simulink model "test_charti"  (R2014a)
settings: Solver=ode45  StartTime=0.0  StopTime=10.0  RelTol=1e-3
settings Model: Creator=simon  LastModifiedBy=simon

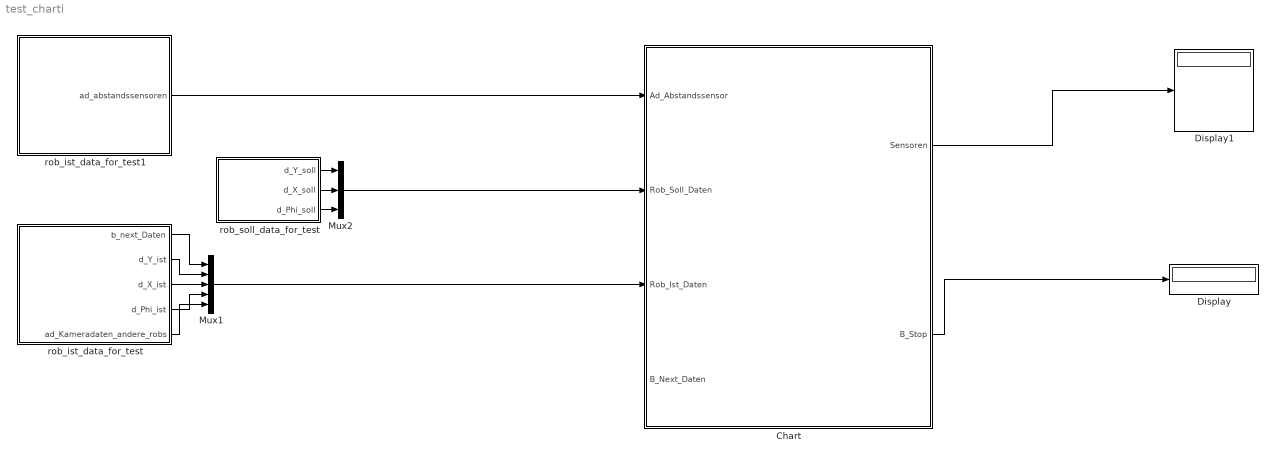
== system test_charti ==
  Chart : Stateflow chart  TreatAsAtomicUnit=on
  Display : Display
  Display1 : Display
  Mux1 : Mux  Inputs=5
  Mux2 : Mux  Inputs=3
  rob_ist_data_for_test : Subsystem
  rob_ist_data_for_test1 : Subsystem
  rob_soll_data_for_test : Subsystem
  wires:
  Mux2/1 -> Chart/2(Rob_Soll_Daten)
  rob_soll_data_for_test/1(d_Y_soll) -> Mux2/1
  rob_soll_data_for_test/2(d_X_soll) -> Mux2/2
  rob_soll_data_for_test/3(d_Phi_soll) -> Mux2/3
  rob_ist_data_for_test/1(b_next_Daten) -> Mux1/1
  rob_ist_data_for_test/2(d_Y_ist) -> Mux1/2
  rob_ist_data_for_test/3(d_X_ist) -> Mux1/3
  rob_ist_data_for_test/4(d_Phi_ist) -> Mux1/4
  rob_ist_data_for_test/5(ad_Kameradaten_andere_robs) -> Mux1/5
  Mux1/1 -> Chart/3(Rob_Ist_Daten)
  rob_ist_data_for_test1/1(ad_abstandssensoren) -> Chart/1(Ad_Abstandssensor)
  Chart/1(Sensoren) -> Display1/1
  Chart/2(B_Stop) -> Display/1

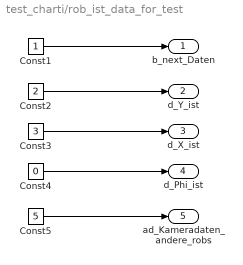
== system test_charti/rob_ist_data_for_test ==
  Const1 : Constant  OutDataTypeStr=double
  Const2 : Constant  Value=2  OutDataTypeStr=double
  Const3 : Constant  Value=3  OutDataTypeStr=double
  Const4 : Constant  Value=0  OutDataTypeStr=double
  Const5 : Constant  Value=5  OutDataTypeStr=double
  b_next_Daten : Outport
  d_Y_ist : Outport  Port=2
  d_X_ist : Outport  Port=3
  d_Phi_ist : Outport  Port=4
  ad_Kameradaten_andere_robs : Outport  Port=5
  wires:
  Const4/1 -> d_Phi_ist/1
  Const3/1 -> d_X_ist/1
  Const1/1 -> b_next_Daten/1
  Const2/1 -> d_Y_ist/1
  Const5/1 -> ad_Kameradaten_andere_robs/1

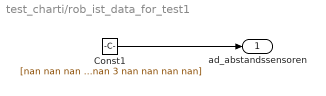
== system test_charti/rob_ist_data_for_test1 ==
  Const1 : Constant  Value=[nan nan nan nan 3 nan nan nan nan]  OutDataTypeStr=double
  ad_abstandssensoren : Outport
  wires:
  Const1/1 -> ad_abstandssensoren/1

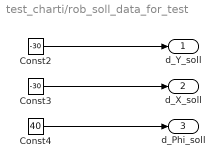
== system test_charti/rob_soll_data_for_test ==
  Const2 : Constant  Value=-30  OutDataTypeStr=double
  Const3 : Constant  Value=-30  OutDataTypeStr=double
  Const4 : Constant  Value=40  OutDataTypeStr=double
  d_Y_soll : Outport
  d_X_soll : Outport  Port=2
  d_Phi_soll : Outport  Port=3
  wires:
  Const4/1 -> d_Phi_soll/1
  Const3/1 -> d_X_soll/1
  Const2/1 -> d_Y_soll/1

== stateflow chart test_charti/Chart ==
  state astern
  state Kollisionsdetektion_state %Kollisionsdetektion
    during: [B_Stop, Sensoren] = kollisionsdetektion(Rob_Ist_Daten, Rob_Soll_Daten, Ad_Abstandssensor)
  state ?
  (default) -> astern
  astern -> Kollisionsdetektion_state %Kollisionsdetektion
  Kollisionsdetektion_state %Kollisionsdetektion -> ? : [B_Stop]
  data: rob_ist_daten function_input; rob_soll_daten function_input; ad_abstandssensor function_input; b_stop function_output; sensoren function_output; Ad_Abstandssensor input; Rob_Soll_Daten input; Rob_Ist_Daten input; Sensoren output; B_Stop output; B_Next_Daten input
  function [b_stop, sensoren]= kollisionsdetektion(rob_ist_daten, rob_soll_daten,ad_abstandssensor):
    | %Version: 0.1
    | %edited: Stall
    | function [b_stop, sensoren]= kollisionsdetektion(rob_ist_daten, rob_soll_daten,ad_abstandssensor)   
    |    sensorreichweite = 1000;                             %Reichweite, die die Sensoren detektieren können
    |    gew_sichtweite = 400;                                %gewünschte Weite die die Sensoren detektieren sollen
    |    
    |    sensoren_fr = [0; 0; 0; 0];                             %Array für die Sensoren in Fahrtrichtung
    |    
    |    %----------------Aufbereiten der eingehenden zusammengefassten Daten------
    |    b_next_Daten = rob_ist_daten(1);
    |    
    |    y_ist = rob_ist_daten(2);
    |    x_ist = rob_ist_daten(3);
    |    phi_ist_grad = rob_ist_daten(4);
    |    
    |    y_soll = rob_soll_daten(1);
    |    x_soll = rob_soll_daten(2);
    |    
    |    % Ist- und Sollkoordinaten in Vektoren
    |    P_ist = [x_ist y_ist];
    |    P_soll = [x_soll y_soll];
    |    
    |    
    |    %-----------------Fahrtrichtungsvektor u. Winkel--------------
    |    V_FR = P_soll - P_ist;                              %Vektor errechnen, der in Fahrtrichtung zeigt
    |    phi_fr_grad = (180/pi) * atan2(V_FR(2),V_FR(1));    %atan2(y,x)! -> gibt gleich korrekten Winkel, atan() gibt nur
    |    %im Wertebereich von -pi/2 bis
    |    %pi/2 zurück
    |    
    |    if phi_fr_grad < 0
    |        phi_fr_grad = phi_fr_grad + 360;                %keine negativen Winkel zulassen
    |    end
    |    
    |    %-----------------Versatz Abstandssensor zu Abstandssensor--------------
    |    phi_vss_grad = 360 / 9;                             %360° bei 9 Sensoren (40 Grad)
    |    
    |    
    |    %-----------------Winkel Zwischen Hauptachse u. Fahrtrichtung--------------
    |    phi_rel_ha_grad = phi_fr_grad - phi_ist_grad;
    |    
    |    if phi_rel_ha_grad < 0
    |        phi_rel_ha_grad = phi_rel_ha_grad + 360;                %keine negativen Winkel zulassen
    |    end
    |    
    |    
    |    %--------------Wähle 4 Sensoren, die der Fahrtrichtung am nächsten---------
    |    
    |    sensor_nr_mit_dezimalstellen = phi_rel_ha_grad / phi_vss_grad;
    |    sensoren_fr(2) = fix(sensor_nr_mit_dezimalstellen) + 1;     %fix: Nachkommastellen abschneiden
    |    sensoren_fr(1) = sensoren_fr(2) - 1;
    |    sensoren_fr(3) = sensoren_fr(2) + 1;
    |    sensoren_fr(4) = sensoren_fr(2) + 2;
    |    
    |    for i = 1 : 1 : max(size(sensoren_fr))
    |        sensoren_fr(i)= pruefe_u_korregiere_sensor_nr(sensoren_fr(i));          %Nummern in Bereich 1_9 überführen
    |    end
    |    
    |    sensoren1 = sensoren_fr(1);
    |    sensoren2 = sensoren_fr(2);
    |    sensoren3 = sensoren_fr(3);
    |    sensoren4 = sensoren_fr(4);
    |    
    |    sensoren = sensoren_fr;  %Nummern der Sensoren die für die Detektion ausgewählt wurden zurückgeben
    |    
    |    if ((ad_abstandssensor(sensoren_fr(1))<gew_sichtweite) || (ad_abstandssensor(sensoren_fr(2))<gew_sichtweite) || ...
    |        (ad_abstandssensor(sensoren_fr(3))<gew_sichtweite) || (ad_abstandssensor(sensoren_fr(4))<gew_sichtweite))
    |        b_stop = true;
    |    else
    |        b_stop = false;
    |    end
    | end
